simulink model "labor11_Sim"  (R2024a)
settings: Solver=VariableStepAuto  StartTime=0.0  StopTime=100  MaxStep=0.1  RelTol=1e-3
values from neighbouring files (symbols this model uses):
  A = [0 1;-k/m -b/m]    [lab_13.m]    (also in labor13.m)
  B = [0;1/m]    [lab_13.m]    (also in labor13.m)
  C = [1 0]    [lab_13.m]    (also in labor13.m)
  G = acker(A', C', [so1 so2])'    [lab_13.m]
  K = acker(A,B,[sc1 sc2])    [lab_13.m]    (also in labor13.m)
  Mu = Mxu(end)    [lab_13.m]    (also in labor13.m)
  Mx = Mxu(1:2)    [lab_13.m]    (also in labor13.m)
libraries: simulink x1
settings Model: Creator=hallgato  LastModifiedBy=Admin

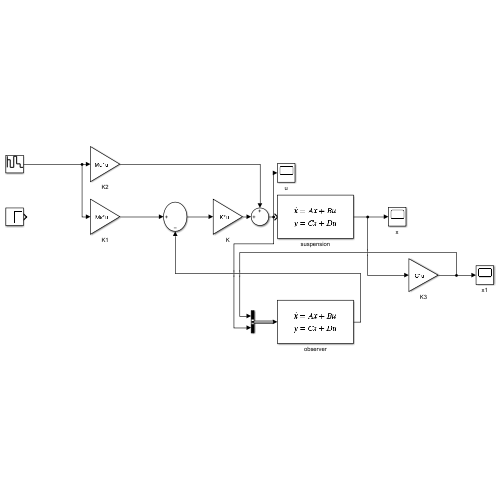
[thumbnail: Simulink's stored preview of the top-level diagram]
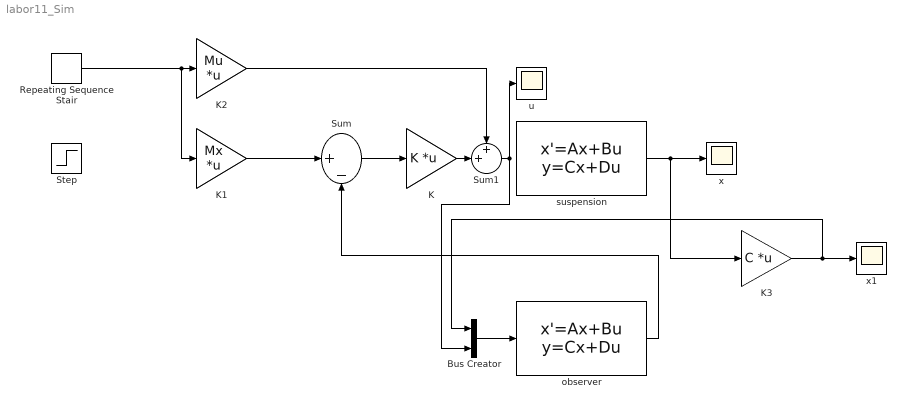
== system labor11_Sim ==
  Bus Creator : BusCreator  Inputs=2
  K : Gain  Gain=K  Multiplication=Matrix(K*u)
  K1 : Gain  Gain=Mx  Multiplication=Matrix(K*u)
  K2 : Gain  Gain=Mu  Multiplication=Matrix(K*u)
  K3 : Gain  Gain=C  Multiplication=Matrix(K*u)
  Repeating Sequence Stair : simulink/Sources/Repeating Sequence Stair  OutValues=[3 1 4 2 1].'  tsamp=20  OutMin=[]  OutMax=[]  OutDataTypeStr=double  OutputDataTypeScalingMode=double  OutDataType=fixdt(0,8)  ConRadixGroup=Best Precision: Vector-wise  OutScaling=2^-12
  Step : Step  After=0.5  SampleTime=0
  Sum : Sum  Inputs=|+-
  Sum1 : Sum  Inputs=++|
  observer : StateSpace  A=A-G*C  B=[G B]  C=eye(2)  D=zeros(2)  InitialCondition=[0 0]
  suspension : StateSpace  A=A  B=B  C=eye(2)  D=zeros(2,1)  InitialCondition=[0.1 0]
  u : Scope
  x : Scope
  x1 : Scope
  wires:
  suspension/1 -> K3/1, x/1
  Sum/1 -> K/1
  K1/1 -> Sum/1
  K/1 -> Sum1/2
  Sum1/1 -> u/1, Bus Creator/2
  K2/1 -> Sum1/1
  Repeating Sequence Stair/1 -> K1/1, K2/1
  observer/1 -> Sum/2
  Bus Creator/1 -> observer/1
  K3/1 -> Bus Creator/1, x1/1
